simulink model "Simulink_group37"  (R2023b)
settings: Solver=FixedStepAuto  StartTime=0.0  StopTime=10.0  FixedStep=1e-3  RelTol=1e-3  EnableMultiTasking=on
undefined symbols (not defined in the file): D0, D1, D10, D11, D12, D13, D2, D3, D4, D5, D6, D7, D8, D9, PTA0, PTA1, PTA2, PTB23, PTB9, PTC16, PTC17, PTC2, PTC3, PTC4, PTD0, PTD1, PTD2, PTD3
libraries: frdmk64flib x15
settings Model: ExtModeTrigDuration=5  Creator=aless  LastModifiedBy=aless
settings OptimizationCC: EnhancedBackFolding=on  PassReuseOutputArgsAs=Individual arguments  ZeroExternalMemoryAtStartup=off  ZeroInternalMemoryAtStartup=off  MaxStackSize=64  OptimizeBlockOrder=speed  DifferentSizesBufferReuse=on  OptimizationCustomize=off  EfficientTunableParamExpr=on
settings DebuggingCC: ParameterTunabilityLossMsg=error
settings HardwareCC: ProdBitPerPointer=32  ProdBitPerSizeT=32  ProdBitPerPtrDiffT=32  ProdLargestAtomicInteger=Long  ProdLargestAtomicFloat=Double  ProdWordSize=32  ProdHWDeviceType=ARM Compatible->ARM Cortex
settings SFSimCC: MATLABDynamicMemAlloc=off
settings RTWCC: Description=Embedded Coder  SystemTargetFile=ert.tlc  HardwareBoard=NXP FRDM-K64F  TLCOptions="-aInlineSetEventsForThisBaseRateFcn=TLC_FALSE -aSuppressMultiTaskScheduler=TLC_FALSE  -aRateBasedStepFcn=0"  TemplateMakefile=ert_default_tmf  Toolchain=GNU Tools for ARM Embedded Processors
settings CodeAppCC: ForceParamTrailComments=on  IgnoreCustomStorageClasses=off  OperatorAnnotations=on  SimulinkDataObjDesc=on  SFDataObjDesc=on  InsertBlockDesc=on
settings ERTTargetCC: ExtModeTransport=4  ExtModeMexFile=sendToCommService

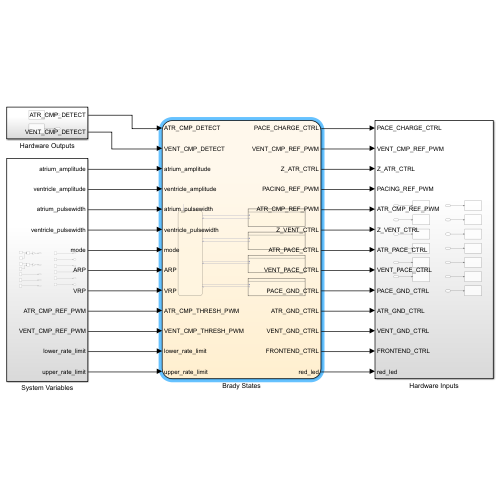
[thumbnail: Simulink's stored preview of the top-level diagram]
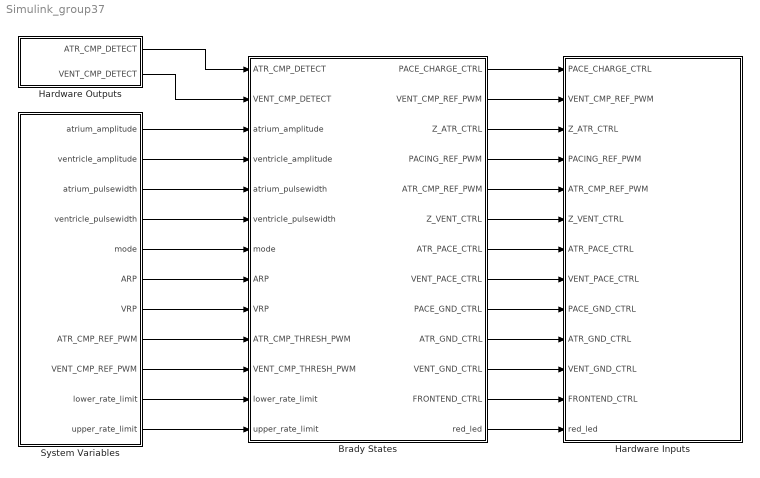
== system Simulink_group37 ==
  Brady States : Stateflow chart  TreatAsAtomicUnit=on
      settings: PortSchema="{\"entries\":[{\"content\":{\"sides\":[{\"content\":{\"connectorIds\":[\"In1\",\"In2\",\"In3\",\"In4\",\"In5\",\"In6\",\"In7\",\"In8\",\"In9\",\"In10\",\"In11\",\"In12\",\"In13\"]},\"type\":\"ConnectorPlacement.EquallySpacedRectSide\",\"uuid\":\"d1839c8f-6221-46d4-ade1-365648b0880c\"},{\"content\":{\"connectorIds\":[\"Out1\",\"Out2\",\"Out3\",\"Out4\",\"Out5\",\"Out6\",\"Out7\",\"Out8\",\"Out9\",\"Out12\",\"Out10\",\"Out11\",\"Out13\"],\"side\":\"RIGHT\"},\"type\":\"ConnectorPlacement.EquallySpacedRectSide\",\"uuid\":\"5469c751-f649-49a4-acaa-2051f4899f66\"},{\"content\":{\"side\":\"TOP\"},\"type\":\"ConnectorPlacement.EquallySpacedRectSide\",\"uuid\":\"ee663bab-8db3-49ac-8698-0304788d9d5e\"}]},\"type\":\"ConnectorPlacement.EquallySpacedConnector\",\"uuid\":\"0582f962-be2e-4f7f-ab84-ab175671d8de\"}],\"packageUris\":[\"http://schema.mathworks.com/mf0/Connector/R2020b\"],\"version\":\"1.0\"}"
  Hardware Inputs : Subsystem
  Hardware Outputs : Subsystem
  System Variables : Subsystem
  wires:
  System Variables/5(mode) -> Brady States/7(mode)
  System Variables/3(atrium_pulsewidth) -> Brady States/5(atrium_pulsewidth)
  System Variables/4(ventricle_pulsewidth) -> Brady States/6(ventricle_pulsewidth)
  System Variables/6(ARP) -> Brady States/8(ARP)
  System Variables/7(VRP) -> Brady States/9(VRP)
  System Variables/8(ATR_CMP_REF_PWM) -> Brady States/10(ATR_CMP_THRESH_PWM)
  System Variables/9(VENT_CMP_REF_PWM) -> Brady States/11(VENT_CMP_THRESH_PWM)
  System Variables/1(atrium_amplitude) -> Brady States/3(atrium_amplitude)
  System Variables/2(ventricle_amplitude) -> Brady States/4(ventricle_amplitude)
  Hardware Outputs/1(ATR_CMP_DETECT) -> Brady States/1(ATR_CMP_DETECT)
  Hardware Outputs/2(VENT_CMP_DETECT) -> Brady States/2(VENT_CMP_DETECT)
  Brady States/1(PACE_CHARGE_CTRL) -> Hardware Inputs/1(PACE_CHARGE_CTRL)
  Brady States/3(Z_ATR_CTRL) -> Hardware Inputs/3(Z_ATR_CTRL)
  Brady States/4(PACING_REF_PWM) -> Hardware Inputs/4(PACING_REF_PWM)
  Brady States/5(ATR_CMP_REF_PWM) -> Hardware Inputs/5(ATR_CMP_REF_PWM)
  Brady States/6(Z_VENT_CTRL) -> Hardware Inputs/6(Z_VENT_CTRL)
  Brady States/7(ATR_PACE_CTRL) -> Hardware Inputs/7(ATR_PACE_CTRL)
  Brady States/8(VENT_PACE_CTRL) -> Hardware Inputs/8(VENT_PACE_CTRL)
  Brady States/9(PACE_GND_CTRL) -> Hardware Inputs/9(PACE_GND_CTRL)
  Brady States/12(ATR_GND_CTRL) -> Hardware Inputs/10(ATR_GND_CTRL)
  Brady States/10(VENT_GND_CTRL) -> Hardware Inputs/11(VENT_GND_CTRL)
  Brady States/11(FRONTEND_CTRL) -> Hardware Inputs/12(FRONTEND_CTRL)
  System Variables/10(lower_rate_limit) -> Brady States/12(lower_rate_limit)
  System Variables/11(upper_rate_limit) -> Brady States/13(upper_rate_limit)
  Brady States/2(VENT_CMP_REF_PWM) -> Hardware Inputs/2(VENT_CMP_REF_PWM)
  Brady States/13(red_led) -> Hardware Inputs/13(red_led)

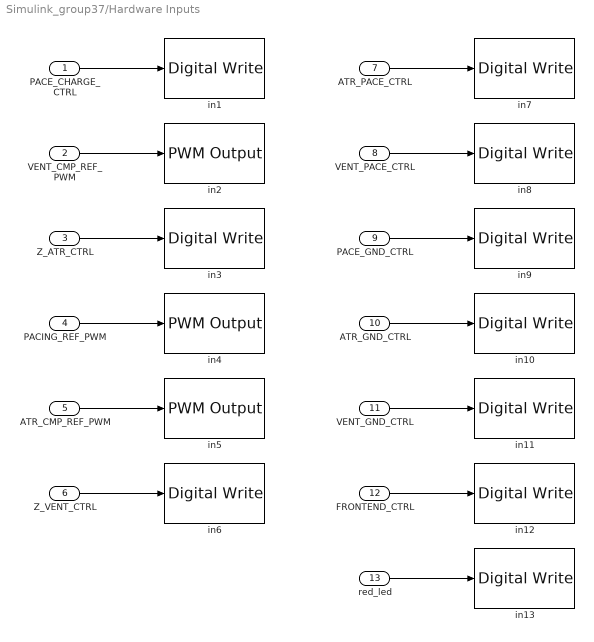
== system Simulink_group37/Hardware Inputs ==
  PACE_CHARGE_CTRL : Inport
  VENT_CMP_REF_PWM : Inport  Port=2
  Z_ATR_CTRL : Inport  Port=3
  PACING_REF_PWM : Inport  Port=4
  ATR_CMP_REF_PWM : Inport  Port=5
  Z_VENT_CTRL : Inport  Port=6
  ATR_PACE_CTRL : Inport  Port=7
  VENT_PACE_CTRL : Inport  Port=8
  PACE_GND_CTRL : Inport  Port=9
  ATR_GND_CTRL : Inport  Port=10
  VENT_GND_CTRL : Inport  Port=11
  FRONTEND_CTRL : Inport  Port=12
  red_led : Inport  Port=13
  in1 : frdmk64flib/Digital Write  Whichpin=PTB9 (D2)
  in10 : frdmk64flib/Digital Write  Whichpin=PTD2 (D11)
  in11 : frdmk64flib/Digital Write  Whichpin=PTD3 (D12)
  in12 : frdmk64flib/Digital Write  Whichpin=PTD1 (D13)
  in13 : frdmk64flib/Digital Write  Whichpin=RED_LED
  in2 : frdmk64flib/PWM Output  Whichpin=PTA1 (D3)  InitialFrequency=2000  InitialDutyCycle=30
  in3 : frdmk64flib/Digital Write  Whichpin=PTB23 (D4)
  in4 : frdmk64flib/PWM Output  Whichpin=PTA2 (D5)  InitialFrequency=2000  InitialDutyCycle=30
  in5 : frdmk64flib/PWM Output  Whichpin=PTC2 (D6)  InitialFrequency=2000  InitialDutyCycle=30
  in6 : frdmk64flib/Digital Write  Whichpin=PTC3 (D7)
  in7 : frdmk64flib/Digital Write  Whichpin=PTA0 (D8)
  in8 : frdmk64flib/Digital Write  Whichpin=PTC4 (D9)
  in9 : frdmk64flib/Digital Write  Whichpin=PTD0 (D10)
  wires:
  ATR_GND_CTRL/1 -> in10/1
  PACING_REF_PWM/1 -> in4/1
  Z_VENT_CTRL/1 -> in6/1
  VENT_GND_CTRL/1 -> in11/1
  VENT_PACE_CTRL/1 -> in8/1
  ATR_CMP_REF_PWM/1 -> in5/1
  FRONTEND_CTRL/1 -> in12/1
  PACE_CHARGE_CTRL/1 -> in1/1
  ATR_PACE_CTRL/1 -> in7/1
  PACE_GND_CTRL/1 -> in9/1
  Z_ATR_CTRL/1 -> in3/1
  VENT_CMP_REF_PWM/1 -> in2/1
  red_led/1 -> in13/1

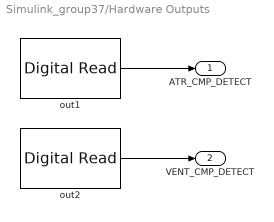
== system Simulink_group37/Hardware Outputs ==
  out1 : frdmk64flib/Digital Read  Whichpin=PTC16 (D0)  SampleTime=-1
  out2 : frdmk64flib/Digital Read  Whichpin=PTC17 (D1)  SampleTime=-1
  ATR_CMP_DETECT : Outport
  VENT_CMP_DETECT : Outport  Port=2
  wires:
  out1/1 -> ATR_CMP_DETECT/1
  out2/1 -> VENT_CMP_DETECT/1

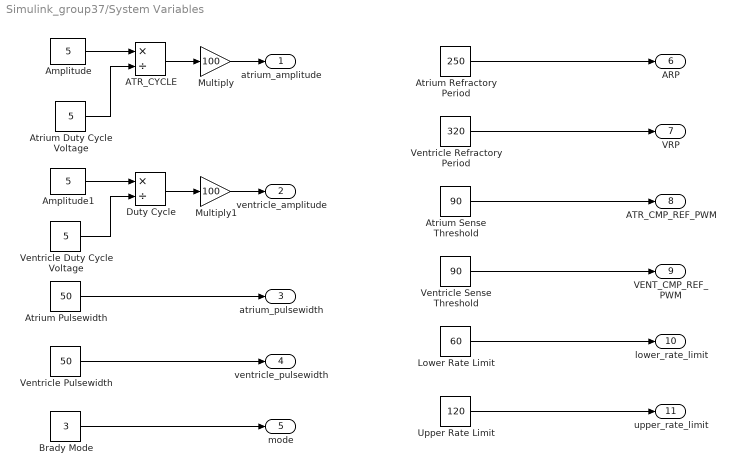
== system Simulink_group37/System Variables ==
  ATR_CYCLE : Product  Inputs=*/
  Amplitude : Constant  Value=5
  Amplitude1 : Constant  Value=5
  Atrium Duty Cycle Voltage : Constant  Value=5
  Atrium Pulsewidth : Constant  Value=50
  Atrium Refractory Period : Constant  Value=250
  Atrium Sense Threshold : Constant  Value=90
  Brady Mode : Constant  Value=3
  Duty Cycle : Product  Inputs=*/
  Lower Rate Limit : Constant  Value=60
  Multiply : Gain  Gain=100
  Multiply1 : Gain  Gain=100
  Upper Rate Limit : Constant  Value=120
  Ventricle Duty Cycle Voltage : Constant  Value=5
  Ventricle Pulsewidth : Constant  Value=50
  Ventricle Refractory Period : Constant  Value=320
  Ventricle Sense Threshold : Constant  Value=90
  atrium_amplitude : Outport
  ventricle_amplitude : Outport  Port=2
  atrium_pulsewidth : Outport  Port=3
  ventricle_pulsewidth : Outport  Port=4
  mode : Outport  Port=5
  ARP : Outport  Port=6
  VRP : Outport  Port=7
  ATR_CMP_REF_PWM : Outport  Port=8
  VENT_CMP_REF_PWM : Outport  Port=9
  lower_rate_limit : Outport  Port=10
  upper_rate_limit : Outport  Port=11
  wires:
  Ventricle Refractory Period/1 -> VRP/1
  Ventricle Pulsewidth/1 -> ventricle_pulsewidth/1
  Atrium Refractory Period/1 -> ARP/1
  Ventricle Sense Threshold/1 -> VENT_CMP_REF_PWM/1
  Atrium Sense Threshold/1 -> ATR_CMP_REF_PWM/1
  Brady Mode/1 -> mode/1
  Atrium Pulsewidth/1 -> atrium_pulsewidth/1
  ATR_CYCLE/1 -> Multiply/1
  Multiply/1 -> atrium_amplitude/1
  Multiply1/1 -> ventricle_amplitude/1
  Duty Cycle/1 -> Multiply1/1
  Amplitude1/1 -> Duty Cycle/1
  Ventricle Duty Cycle Voltage/1 -> Duty Cycle/2
  Amplitude/1 -> ATR_CYCLE/1
  Atrium Duty Cycle Voltage/1 -> ATR_CYCLE/2
  Lower Rate Limit/1 -> lower_rate_limit/1
  Upper Rate Limit/1 -> upper_rate_limit/1

== stateflow chart Simulink_group37/Brady States ==
  state AOO [group]
    state Discharging
      entry:
      %discharge C22
      %charge C21
      PACE_CHARGE_CTRL = false
      PACE_GND_CTRL = true
      ATR_PACE_CTRL = true
      ATR_GND_CTRL = false
      Z_ATR_CTRL = false
      Z_VENT_CTRL = false
      VENT_GND_CTRL = false
      VENT_PACE_CTRL  = false
      red_led=true %for testing
    state Charging
      entry:
      %charge C22
      ATR_PACE_CTRL = false
      VENT_PACE_CTRL = false
      PACING_REF_PWM = atrium_amplitude
      PACE_CHARGE_CTRL = true
      %discharge C21 into atrium
      PACE_GND_CTRL = true
      VENT_PACE_CTRL = false
      Z_ATR_CTRL = false
      Z_VENT_CTRL = false
      ATR_PACE_CTRL = false
      ATR_GND_CTRL = true
      VENT_GND_CTRL = false
      red_led=false %for testing
    AOO.Charging -> AOO.Discharging [order 1] : [after(((60000/lower_rate_limit)-atrium_pulsewidth),msec)]
    AOO.Discharging -> AOO.Charging : [after((atrium_pulsewidth),msec)]
  state Mode
  state VOO [group]
    state Charging
      entry:
      %charge C22
      ATR_PACE_CTRL = false
      VENT_PACE_CTRL = false
      PACING_REF_PWM = ventricle_amplitude
      PACE_CHARGE_CTRL = true
      %discharge C21 into ventricle ground
      PACE_GND_CTRL = true
      VENT_PACE_CTRL = false
      Z_ATR_CTRL = false
      Z_VENT_CTRL = false
      ATR_PACE_CTRL = false
      ATR_GND_CTRL = false
      VENT_GND_CTRL = true
      red_led=false
    state Discharging
      entry:
      %discharge C22 to charge C21
      PACE_CHARGE_CTRL = false
      PACE_GND_CTRL = true
      ATR_PACE_CTRL = false
      ATR_GND_CTRL = false
      Z_VENT_CTRL = false
      Z_ATR_CTRL = false
      VENT_GND_CTRL = false
      VENT_PACE_CTRL = true
      red_led=true
    VOO.Charging -> VOO.Discharging [order 1] : [after(((60000/lower_rate_limit)-ventricle_pulsewidth),msec)]
    VOO.Discharging -> VOO.Charging : [after((ventricle_pulsewidth),msec)]
  state AAI [group]
    state Charging
      entry:
      %sensing
      FRONTEND_CTRL = true
      ATR_CMP_REF_PWM = ATR_CMP_THRESH_PWM
      %charge C22
      ATR_PACE_CTRL = false
      VENT_PACE_CTRL = false
      PACING_REF_PWM = atrium_amplitude
      PACE_CHARGE_CTRL = true
      %discharge C21 into atrium
      PACE_GND_CTRL = true
      VENT_PACE_CTRL = false
      Z_ATR_CTRL = false
      Z_VENT_CTRL = false
      ATR_PACE_CTRL = false
      ATR_GND_CTRL = true
      VENT_GND_CTRL = false
    state Discharging
      entry:
      %discharge C22 to charge C21
      PACE_CHARGE_CTRL = false
      PACE_GND_CTRL = true
      VENT_PACE_CTRL = false
      VENT_GND_CTRL = false
      Z_VENT_CTRL = false
      Z_ATR_CTRL = false
      ATR_GND_CTRL = false
      ATR_PACE_CTRL = true
    state Transition
      %check for sensing
      FRONTEND_CTRL = true
    AAI.Discharging -> AAI.Charging : [after(atrium_pulsewidth, msec)]
    AAI.Charging -> AAI.Transition [order 1] : [after(ARP, msec)]
    AAI.Transition -> AAI.Discharging [order 2] : [after(((60000/lower_rate_limit)-atrium_pulsewidth-ARP),msec)]
    AAI.Transition -> AAI.Charging [order 1] : [ATR_CMP_DETECT == true]
  state VVI [group]
    state Charging
      entry:
      %sensing
      FRONTEND_CTRL = true
      VENT_CMP_REF_PWM = VENT_CMP_THRESH_PWM
      %charge C22
      ATR_PACE_CTRL = false
      VENT_PACE_CTRL = false
      PACING_REF_PWM = ventricle_amplitude
      PACE_CHARGE_CTRL = true
      %Discharge C21 into ventricle
      PACE_GND_CTRL = true
      VENT_PACE_CTRL = false
      Z_ATR_CTRL = false
      Z_VENT_CTRL = false
      ATR_PACE_CTRL = false
      ATR_GND_CTRL = false
      VENT_GND_CTRL = true
    state Discharging
      entry:
      %discharge C22 to charge C21
      PACE_CHARGE_CTRL = false
      PACE_GND_CTRL = true
      ATR_PACE_CTRL = false
      ATR_GND_CTRL = false
      Z_VENT_CTRL = false
      Z_ATR_CTRL = false
      VENT_GND_CTRL = false
      VENT_PACE_CTRL = true
    state Transition
      %check for sense
      FRONTEND_CTRL = true
    VVI.Discharging -> VVI.Charging : [after(ventricle_pulsewidth, msec)]
    VVI.Charging -> VVI.Transition [order 1] : [after(VRP, msec)]
    VVI.Transition -> VVI.Discharging [order 2] : [after(((60000/lower_rate_limit)-ventricle_pulsewidth-VRP),msec)]
    VVI.Transition -> VVI.Charging [order 1] : [VENT_CMP_DETECT == true]
  Mode -> VVI.Charging [order 4] : [mode==3]
  VVI.Charging -> Mode [order 2] : [mode~=3]
  AAI.Charging -> Mode [order 2] : [mode~=2]
  VOO.Charging -> Mode [order 2] : [mode~=1]
  AOO.Charging -> Mode [order 2] : [mode~=0]
  Mode -> AAI.Charging [order 3] : [mode==2]
  Mode -> VOO.Charging [order 2] : [mode==1]
  Mode -> AOO.Charging [order 1] : [mode==0]
  (default) -> Mode
  data: ATR_CMP_DETECT input; VENT_CMP_DETECT input; atrium_amplitude input; ventricle_amplitude input; atrium_pulsewidth input; ventricle_pulsewidth input; mode input; ARP input; VRP input; ATR_CMP_THRESH_PWM input; VENT_CMP_THRESH_PWM input; PACE_CHARGE_CTRL output; VENT_CMP_REF_PWM output; Z_ATR_CTRL output; PACING_REF_PWM output; ATR_CMP_REF_PWM output; Z_VENT_CTRL output; ATR_PACE_CTRL output; VENT_PACE_CTRL output; PACE_GND_CTRL output; VENT_GND_CTRL output; FRONTEND_CTRL output; ATR_GND_CTRL output; lower_rate_limit input; upper_rate_limit input; red_led output
